simulink model "simulink_puma_robot"  (R2016a)
settings: Solver=VariableStepAuto  StartTime=0.0  StopTime=10  FixedStep=0.3  RelTol=1e-3
settings Model: Creator=84360  LastModifiedBy=user

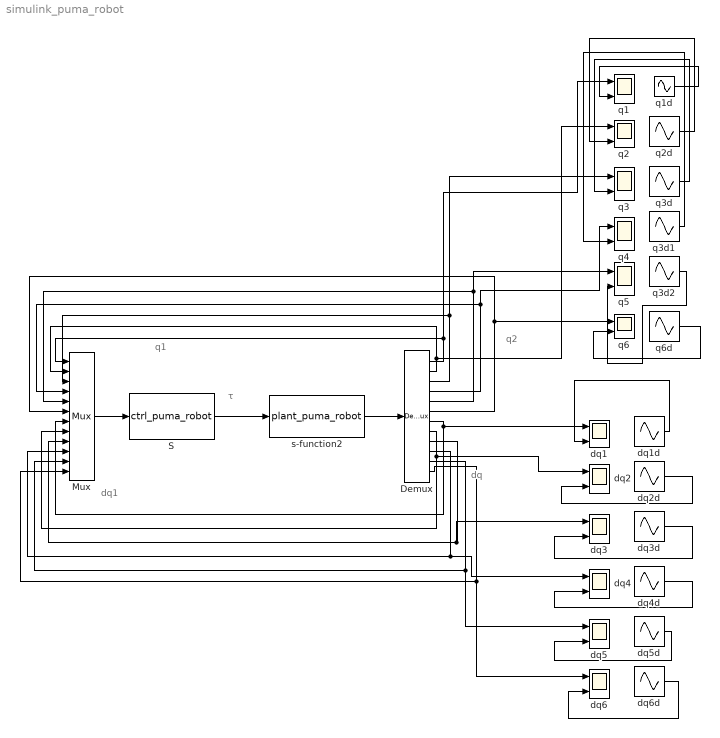
== system simulink_puma_robot ==
  note: q2
  note: dq
  note: τ
  note: dq1
  note: q1
  Demux : Demux  Outputs=12
  Mux : Mux  Inputs=12
  "S " : S-Function  FunctionName=ctrl_puma_robot  SFunctionDeploymentMode=off  EnableBusSupport=off
  dq{1..6} (6 alike) : Scope  NumInputPorts=2
  dq1d : Sin  Amplitude=-pi  Frequency=pi  SampleTime=0
  dq2d : Sin  Amplitude=pi/2  Frequency=pi/2  Phase=pi/2  SampleTime=0
  dq3d : Sin  Amplitude=pi  Frequency=pi  Phase=pi/2  SampleTime=0
  dq4d : Sin  Amplitude=pi  Frequency=pi  Phase=pi/2  SampleTime=0
  dq5d : Sin  Amplitude=-pi  Frequency=pi  SampleTime=0
  dq6d : Sin  Amplitude=-pi/2  Frequency=pi/2  SampleTime=0
  q{1..6} (6 alike) : Scope  NumInputPorts=2
  q1d : Sin  Frequency=pi  Phase=pi/2  SampleTime=0
  q2d : Sin  Frequency=pi/2  SampleTime=0
  q3d : Sin  Frequency=pi  SampleTime=0
  q3d1 : Sin  Frequency=pi  SampleTime=0
  q3d2 : Sin  Frequency=pi  Phase=pi/2  SampleTime=0
  "q6d " : Sin  Frequency=pi/2  Phase=pi/2  SampleTime=0
  "s-function2 " : S-Function  FunctionName=plant_puma_robot  SFunctionDeploymentMode=off  EnableBusSupport=off
  wires:
  Mux/1 -> "S "/1
  "s-function2 "/1 -> Demux/1
  "S "/1 -> "s-function2 "/1
  Demux/1 -> q1/1, Mux/1
  Demux/2 -> q2/1, Mux/2
  Demux/3 -> q3/1, Mux/3
  Demux/4 -> q4/1, Mux/4
  Demux/5 -> q5/1, Mux/5
  Demux/6 -> Mux/6, q6/1
  Demux/7 -> Mux/7, dq1/1
  Demux/8 -> dq2/1, Mux/8
  Demux/9 -> dq3/1, Mux/9
  Demux/10 -> Mux/10, dq4/1
  Demux/11 -> Mux/11, dq5/1
  Demux/12 -> dq6/1, Mux/12
  q1d/1 -> q1/2
  q2d/1 -> q2/2
  q3d/1 -> q3/2
  "q6d "/1 -> q6/2
  dq1d/1 -> dq1/2
  dq6d/1 -> dq6/2
  q3d1/1 -> q4/2
  q3d2/1 -> q5/2
  dq2d/1 -> dq2/2
  dq3d/1 -> dq3/2
  dq4d/1 -> dq4/2
  dq5d/1 -> dq5/2
